simulink model "cart_pole_nonlinear"  (R2024b)
settings: Solver=VariableStepAuto  StartTime=0.0  StopTime=T_sim  RelTol=1e-3
values from neighbouring files (symbols this model uses):
  g = params.g    [cart_pole.m]    (also in cart_pole_v2.m = 9.81)
  J = 0.006767    [cart_pole_v2.m]
  l = params.l    [cart_pole.m]    (also in cart_pole_v2.m = 0.0675)
  m = params.m    [cart_pole.m]    (also in cart_pole_v2.m = 0.69)
  M = params.M    [cart_pole.m]    (also in cart_pole_v2.m = 0.27)
  theta_ref = params.theta_ref    [cart_pole.m]    (also in cart_pole_v2.m = 0)
  X_0 = [deg2rad(5); 0; 0; 0]    [cart_pole.m]    (also in cart_pole_v2.m = [0; 0; deg2rad(5); 0])
libraries: slpidlib x1, simulink_extras x1
settings Model: Creator=martinhaugen  LastModifiedBy=martinhaugen

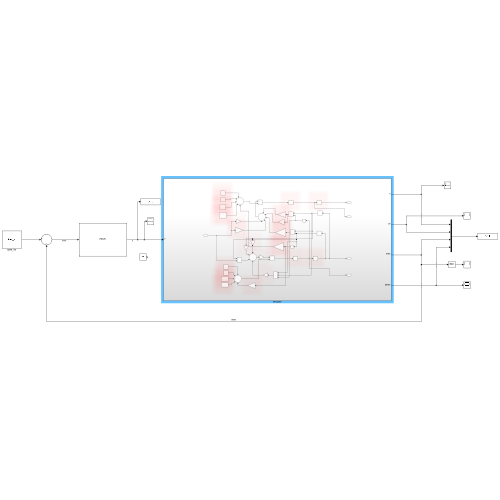
[thumbnail: Simulink's stored preview of the top-level diagram]
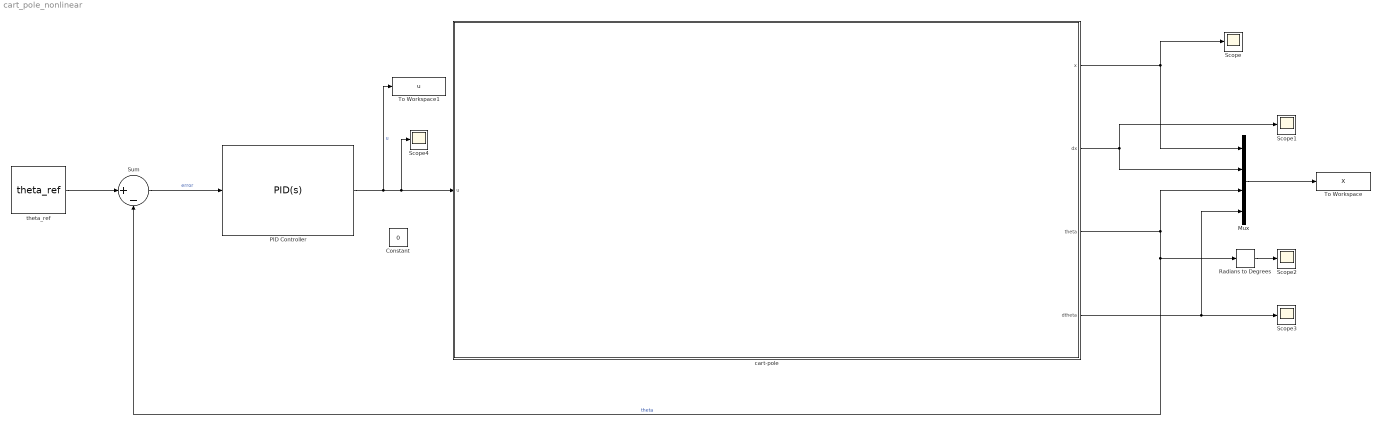
== system cart_pole_nonlinear ==
  Constant : Constant  Value=0
  Mux : Mux
  PID Controller : slpidlib/PID Controller  Controller=PID  Form=Parallel  TimeDomain=Continuous-time  UseExternalTs=off  SampleTime=-1  IntegratorMethod=Forward Euler  FilterMethod=Forward Euler  ControllerParametersSource=internal  P=414.8  I=2449  UseKiTs=off  D=17.56  UseExternalDerivativeSource=off  N=100  UseFilter=on  TunerSelectOption=Transfer Function Based (PID Tuner App)  InitialConditionSource=internal  InitialConditionForIntegrator=0  InitialConditionForFilter=0  DifferentiatorICPrevScaledInput=0  ExternalReset=none  TrackingMode=off  Kt=1  LimitOutput=off  SatLimitsSource=internal  UpperSaturationLimit=inf  LowerSaturationLimit=-inf  LinearizeAsGain=on  AntiWindupMode=none  Kb=1  LimitIntegrator=off  UpperIntegratorSaturationLimit=inf  LowerIntegratorSaturationLimit=-inf  POutMin=[]  POutMax=[]  IOutMin=[]  IOutMax=[]  DOutMin=[]  DOutMax=[]  NOutMin=[]  NOutMax=[]  SumOutMin=[]  SumOutMax=[]  SaturationOutMin=[]  SaturationOutMax=[]  PParamMin=[]  PParamMax=[]  IParamMin=[]  IParamMax=[]  DParamMin=[]  DParamMax=[]  NParamMin=[]  NParamMax=[]  KbParamMin=[]  KbParamMax=[]  KtParamMin=[]  KtParamMax=[]  KbOutMin=[]  KbOutMax=[]  KtOutMin=[]  KtOutMax=[]  IntegratorOutMin=[]  IntegratorOutMax=[]  FilterOutMin=[]  FilterOutMax=[]  SumI1OutMin=[]  SumI1OutMax=[]  SumI2OutMin=[]  SumI2OutMax=[]  SumI3OutMin=[]  SumI3OutMax=[]  SumI4OutMin=[]  SumI4OutMax=[]  SumDOutMin=[]  SumDOutMax=[]  DifferentiatorOutMin=[]  DifferentiatorOutMax=[]  FilterDiffOutCoefMin=[]  FilterDiffOutCoefMax=[]  ReciprocalOutMin=[]  ReciprocalOutMax=[]  SumDenOutMin=[]  SumDenOutMax=[]  SumNumOutMin=[]  SumNumOutMax=[]  DivideOutMin=[]  DivideOutMax=[]  UdiffTsProdOutMin=[]  UdiffTsProdOutMax=[]  NTsProdOutMin=[]  NTsProdOutMax=[]  UintegralTsProdOutMin=[]  UintegralTsProdOutMax=[]  UngainTsProdOutMin=[]  UngainTsProdOutMax=[]  ClampingZeroOutDataTypeStr=Inherit: Inherit via back propagation  ClampingZeroOutMin=[]  ClampingZeroOutMax=[]  FilterDenConstantOutDataTypeStr=Inherit: Inherit via back propagation  FilterDenConstantOutMin=[]  FilterDenConstantOutMax=[]  PCopyOutDataTypeStr=Inherit: Inherit via back propagation  PCopyOutMin=[]  PCopyOutMax=[]  NCopyOutDataTypeStr=Inherit: Inherit via back propagation  NCopyOutMin=[]  NCopyOutMax=[]  IntegratorContinuousStateAttributes=''  IntegratorStateMustResolveToSignalObject=off  IntegratorRTWStateStorageClass=Auto  FilterContinuousStateAttributes=''  FilterStateMustResolveToSignalObject=off  FilterRTWStateStorageClass=Auto  ParallelPVariant=InternalParameters  IdealPVariant=Disabled  IVariant=InternalParameters  DVariant=InternalParameters  IntegratorVariant=Continuous  SatVariant=Disabled  AWVariant=Passthrough  PCopyVariant=Disabled  TRVariant=Disabled  FdbkBlocksVariant=Forward  IdealPFdbkVariant=Disabled  SatFdbkVariant=Disabled  DerivativeFilterVariant=ContFilter  NVariant=InternalParameters  NCopyVariant=Disabled  FilterICVariant=InternalICsFilter  IntegratorICVariant=InternalICs  ExternalResetVariant=Disabled  TRSumVariant=Passthrough  SumFdbkVariant=Disabled  SumVariant=Sum_PID  TsampFilterVariant=InternalTs  TsampNgainVariant=Passthrough  TsampIntegralVariant=Disabled_SignalSpec  ExternalSaturationOutDataTypeStr=Inherit: Same as second input  DerivativeSourceVariant=ErrorSignal  PreIntVariant=InternalPreInt
  Radians to Degrees : simulink_extras/Transformations/Radians to Degrees
  Scope{,1..4} (5 alike) : Scope
  Sum : Sum  Inputs=|+-
  To Workspace : ToWorkspace  VariableName=X  SaveFormat=Timeseries  SampleTime=-1
  To Workspace1 : ToWorkspace  VariableName=u  SaveFormat=Timeseries  SampleTime=-1
  cart-pole : Subsystem
  theta_ref : Constant  Value=theta_ref
  wires:
  PID Controller/1 -> To Workspace1/1, cart-pole/1(u), Scope4/1  "u"
  theta_ref/1 -> Sum/1
  Sum/1 -> PID Controller/1  "error"
  cart-pole/1(x) -> Scope/1, Mux/1
  cart-pole/2(dx) -> Mux/2, Scope1/1
  cart-pole/3(theta) -> Sum/2, Radians to Degrees/1, Mux/3  "theta"
  cart-pole/4(dtheta) -> Scope3/1, Mux/4
  Mux/1 -> To Workspace/1
  Radians to Degrees/1 -> Scope2/1

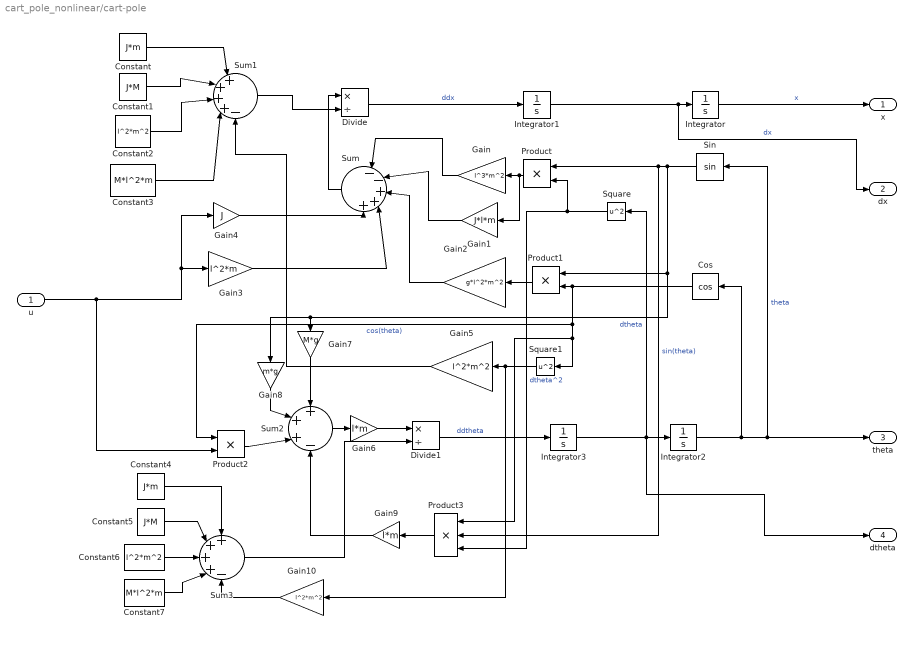
== system cart_pole_nonlinear/cart-pole ==
  u : Inport
  Constant : Constant  Value=J*m
  Constant1 : Constant  Value=J*M
  Constant2 : Constant  Value=l^2*m^2
  Constant3 : Constant  Value=M*l^2*m
  Constant4 : Constant  Value=J*m
  Constant5 : Constant  Value=J*M
  Constant6 : Constant  Value=l^2*m^2
  Constant7 : Constant  Value=M*l^2*m
  Cos : Trigonometry  Operator=cos
  Divide : Product  Inputs=*/
  Divide1 : Product  Inputs=*/
  Gain : Gain  Gain=l^3*m^2
  Gain1 : Gain  Gain=J*l*m
  Gain10 : Gain  Gain=l^2*m^2
  Gain2 : Gain  Gain=g*l^2*m^2
  Gain3 : Gain  Gain=l^2*m
  Gain4 : Gain  Gain=J
  Gain5 : Gain  Gain=l^2*m^2
  Gain6 : Gain  Gain=l*m
  Gain7 : Gain  Gain=M*g
  Gain8 : Gain  Gain=m*g
  Gain9 : Gain  Gain=l*m
  Integrator : Integrator  InitialCondition=X_0(1)
  Integrator1 : Integrator  InitialCondition=X_0(2)
  Integrator2 : Integrator  InitialCondition=X_0(3)
  Integrator3 : Integrator  InitialCondition=X_0(4)
  Product : Product
  Product1 : Product
  Product2 : Product
  Product3 : Product  Inputs=3
  Sin : Trigonometry
  Square : Math  Operator=square
  Square1 : Math  Operator=square
  Sum : Sum  Inputs=|-|-|+|+|+
  Sum1 : Sum  Inputs=|+|+|+|+|-
  Sum2 : Sum  Inputs=+|+|+|-
  Sum3 : Sum  Inputs=+|+|+|+|-
  x : Outport
  dx : Outport  Port=2
  theta : Outport  Port=3
  dtheta : Outport  Port=4
  wires:
  Integrator1/1 -> dx/1, Integrator/1  "dx"
  Integrator/1 -> x/1  "x"
  Divide/1 -> Integrator1/1  "ddx"
  Integrator3/1 -> Integrator2/1, Square/1, dtheta/1  "dtheta"
  Integrator2/1 -> theta/1, Sin/1, Cos/1  "theta"
  Sin/1 -> Product/1, Product3/2, Product1/1, Gain8/1, Gain7/1  "sin(theta)"
  Square/1 -> Product3/3, Product/2  "dtheta^2"
  Product/1 -> Gain1/1, Gain/1
  Gain/1 -> Sum/1
  Gain1/1 -> Sum/2
  Cos/1 -> Product3/1, Square1/1, Product2/1, Product1/2  "cos(theta)"
  Product1/1 -> Gain2/1
  Gain2/1 -> Sum/3
  u/1 -> Gain4/1, Gain3/1, Product2/2
  Gain3/1 -> Sum/4
  Gain4/1 -> Sum/5
  Sum/1 -> Divide/1
  Constant/1 -> Sum1/1
  Constant1/1 -> Sum1/2
  Constant2/1 -> Sum1/3
  Constant3/1 -> Sum1/4
  Square1/1 -> Gain10/1, Gain5/1
  Gain5/1 -> Sum1/5
  Sum1/1 -> Divide/2
  Gain6/1 -> Divide1/1
  Sum2/1 -> Gain6/1
  Gain7/1 -> Sum2/1
  Gain8/1 -> Sum2/2
  Product2/1 -> Sum2/3
  Product3/1 -> Gain9/1
  Gain9/1 -> Sum2/4
  Constant4/1 -> Sum3/1
  Constant5/1 -> Sum3/2
  Constant6/1 -> Sum3/3
  Constant7/1 -> Sum3/4
  Sum3/1 -> Divide1/2
  Gain10/1 -> Sum3/5
  Divide1/1 -> Integrator3/1  "ddtheta"
